simulink model "PA_PUC7_ThreeSystem"  (R2023b)
settings: Solver=ode23  StartTime=0.0  StopTime=7  MaxStep=1e-5  MinStep=1e-6  RelTol=1e-3
libraries: simulink x33, spsSeriesRLCBranchLib x30, spsIGBTDiodeLib x24, spsDiodeLib x21, dspstat3 x18, spsCurrentMeasurementLib x12, spsVoltageMeasurementLib x12, spsMosfetLib x9, spsVariableResistorLib x3, spsDCVoltageSourceLib x3, fuzblock x2, spspowerguiLib x1
settings Model: Creator=T5610  LastModifiedBy=afuaf
settings SolverCC: AlgebraicLoopSolver=TrustRegion
settings DataIOCC: ReturnWorkspaceOutputs=off
settings DebuggingCC: UnconnectedInputMsg=warning  UnconnectedOutputMsg=warning  UnconnectedLineMsg=warning
settings ModelReferenceCC: EnableRefExpFcnMdlSchedulingChecks=on

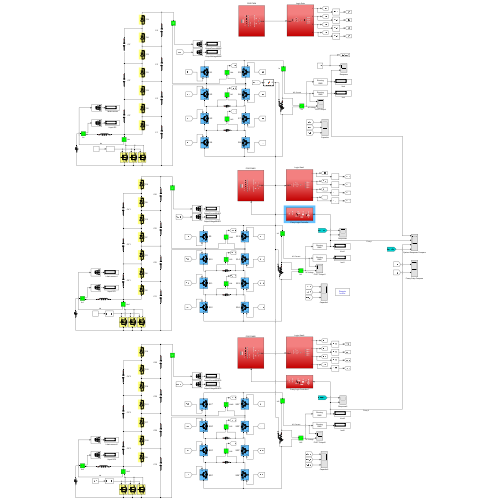
[thumbnail: Simulink's stored preview of the top-level diagram]
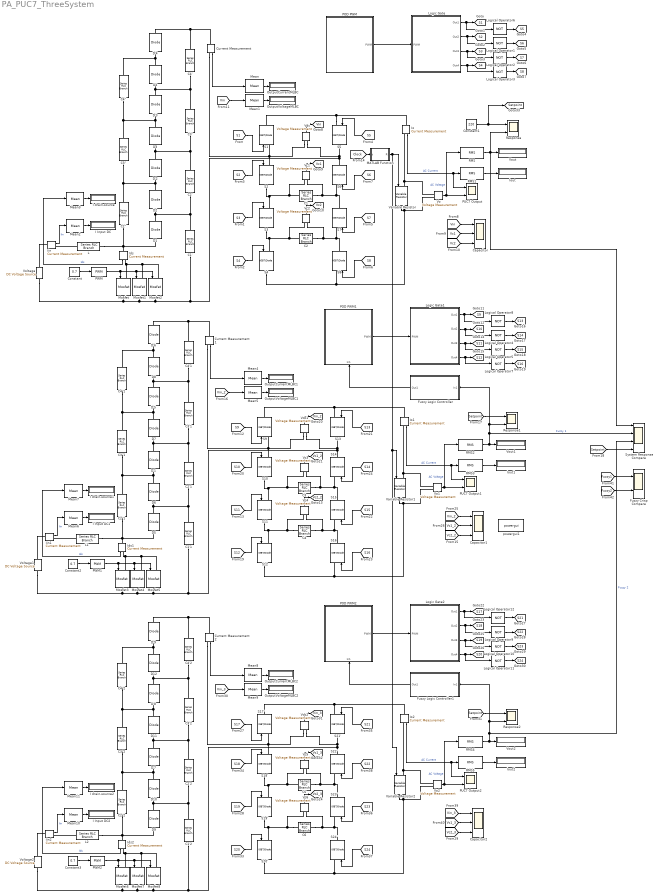
== system PA_PUC7_ThreeSystem ==
  C{1..6} (6 alike) : spsSeriesRLCBranchLib/Series RLC Branch  LConnTagsString=__new0  RConnTagsString=__new0  BranchType=C  Resistance=1  Inductance=100e-03  SetiL0=off  InitialCurrent=0  Capacitance=470e-6  Setx0=on  InitialVoltage=0  Measurements=None
  C1' : spsSeriesRLCBranchLib/Series RLC Branch  LConnTagsString=__new0  RConnTagsString=__new0  BranchType=C  Resistance=5e-3  Inductance=1e-3  SetiL0=off  InitialCurrent=0  Capacitance=3300e-6  Setx0=on  InitialVoltage=0  Measurements=None
  C1'1 : spsSeriesRLCBranchLib/Series RLC Branch  LConnTagsString=__new0  RConnTagsString=__new0  BranchType=C  Resistance=5e-3  Inductance=1e-3  SetiL0=off  InitialCurrent=0  Capacitance=3300e-6  Setx0=on  InitialVoltage=0  Measurements=None
  C1'2 : spsSeriesRLCBranchLib/Series RLC Branch  LConnTagsString=__new0  RConnTagsString=__new0  BranchType=C  Resistance=5e-3  Inductance=1e-3  SetiL0=off  InitialCurrent=0  Capacitance=3300e-6  Setx0=on  InitialVoltage=0  Measurements=None
  C2' : spsSeriesRLCBranchLib/Series RLC Branch  LConnTagsString=__new0  RConnTagsString=__new0  BranchType=C  Resistance=5e-3  Inductance=1e-3  SetiL0=off  InitialCurrent=0  Capacitance=3300e-6  Setx0=on  InitialVoltage=0  Measurements=None
  C2'' : spsSeriesRLCBranchLib/Series RLC Branch  LConnTagsString=__new0  RConnTagsString=__new0  BranchType=C  Resistance=5e-3  Inductance=1e-3  SetiL0=off  InitialCurrent=0  Capacitance=3300e-6  Setx0=on  InitialVoltage=0  Measurements=None
  C2''1 : spsSeriesRLCBranchLib/Series RLC Branch  LConnTagsString=__new0  RConnTagsString=__new0  BranchType=C  Resistance=5e-3  Inductance=1e-3  SetiL0=off  InitialCurrent=0  Capacitance=3300e-6  Setx0=on  InitialVoltage=0  Measurements=None
  C2''2 : spsSeriesRLCBranchLib/Series RLC Branch  LConnTagsString=__new0  RConnTagsString=__new0  BranchType=C  Resistance=5e-3  Inductance=1e-3  SetiL0=off  InitialCurrent=0  Capacitance=3300e-6  Setx0=on  InitialVoltage=0  Measurements=None
  C2'1 : spsSeriesRLCBranchLib/Series RLC Branch  LConnTagsString=__new0  RConnTagsString=__new0  BranchType=C  Resistance=5e-3  Inductance=1e-3  SetiL0=off  InitialCurrent=0  Capacitance=3300e-6  Setx0=on  InitialVoltage=0  Measurements=None
  C2'2 : spsSeriesRLCBranchLib/Series RLC Branch  LConnTagsString=__new0  RConnTagsString=__new0  BranchType=C  Resistance=5e-3  Inductance=1e-3  SetiL0=off  InitialCurrent=0  Capacitance=3300e-6  Setx0=on  InitialVoltage=0  Measurements=None
  C3' : spsSeriesRLCBranchLib/Series RLC Branch  LConnTagsString=__new0  RConnTagsString=__new0  BranchType=C  Resistance=5e-3  Inductance=1e-3  SetiL0=off  InitialCurrent=0  Capacitance=3300e-6  Setx0=on  InitialVoltage=0  Measurements=None
  C3'' : spsSeriesRLCBranchLib/Series RLC Branch  LConnTagsString=__new0  RConnTagsString=__new0  BranchType=C  Resistance=5e-3  Inductance=1e-3  SetiL0=off  InitialCurrent=0  Capacitance=3300e-6  Setx0=on  InitialVoltage=0  Measurements=None
  C3''1 : spsSeriesRLCBranchLib/Series RLC Branch  LConnTagsString=__new0  RConnTagsString=__new0  BranchType=C  Resistance=5e-3  Inductance=1e-3  SetiL0=off  InitialCurrent=0  Capacitance=3300e-6  Setx0=on  InitialVoltage=0  Measurements=None
  C3''2 : spsSeriesRLCBranchLib/Series RLC Branch  LConnTagsString=__new0  RConnTagsString=__new0  BranchType=C  Resistance=5e-3  Inductance=1e-3  SetiL0=off  InitialCurrent=0  Capacitance=3300e-6  Setx0=on  InitialVoltage=0  Measurements=None
  C3'1 : spsSeriesRLCBranchLib/Series RLC Branch  LConnTagsString=__new0  RConnTagsString=__new0  BranchType=C  Resistance=5e-3  Inductance=1e-3  SetiL0=off  InitialCurrent=0  Capacitance=3300e-6  Setx0=on  InitialVoltage=0  Measurements=None
  C3'2 : spsSeriesRLCBranchLib/Series RLC Branch  LConnTagsString=__new0  RConnTagsString=__new0  BranchType=C  Resistance=5e-3  Inductance=1e-3  SetiL0=off  InitialCurrent=0  Capacitance=3300e-6  Setx0=on  InitialVoltage=0  Measurements=None
  C4' : spsSeriesRLCBranchLib/Series RLC Branch  LConnTagsString=__new0  RConnTagsString=__new0  BranchType=C  Resistance=5e-3  Inductance=1e-3  SetiL0=off  InitialCurrent=0  Capacitance=3300e-6  Setx0=on  InitialVoltage=0  Measurements=None
  C4'' : spsSeriesRLCBranchLib/Series RLC Branch  LConnTagsString=__new0  RConnTagsString=__new0  BranchType=C  Resistance=5e-3  Inductance=1e-3  SetiL0=off  InitialCurrent=0  Capacitance=3300e-6  Setx0=on  InitialVoltage=0  Measurements=None
  C4''1 : spsSeriesRLCBranchLib/Series RLC Branch  LConnTagsString=__new0  RConnTagsString=__new0  BranchType=C  Resistance=5e-3  Inductance=1e-3  SetiL0=off  InitialCurrent=0  Capacitance=3300e-6  Setx0=on  InitialVoltage=0  Measurements=None
  C4''2 : spsSeriesRLCBranchLib/Series RLC Branch  LConnTagsString=__new0  RConnTagsString=__new0  BranchType=C  Resistance=5e-3  Inductance=1e-3  SetiL0=off  InitialCurrent=0  Capacitance=3300e-6  Setx0=on  InitialVoltage=0  Measurements=None
  C4'1 : spsSeriesRLCBranchLib/Series RLC Branch  LConnTagsString=__new0  RConnTagsString=__new0  BranchType=C  Resistance=5e-3  Inductance=1e-3  SetiL0=off  InitialCurrent=0  Capacitance=3300e-6  Setx0=on  InitialVoltage=0  Measurements=None
  C4'2 : spsSeriesRLCBranchLib/Series RLC Branch  LConnTagsString=__new0  RConnTagsString=__new0  BranchType=C  Resistance=5e-3  Inductance=1e-3  SetiL0=off  InitialCurrent=0  Capacitance=3300e-6  Setx0=on  InitialVoltage=0  Measurements=None
  Capacitor : Scope  NumInputPorts=3
  Capacitor1 : Scope  NumInputPorts=3
  Capacitor2 : Scope  NumInputPorts=3
  Constant : Constant  Value=0.7
  Constant1 : Constant  Value=220
  Constant2 : Constant  Value=0.7
  Constant3 : Constant  Value=0.7
  Current Measurement : spsCurrentMeasurementLib/Current Measurement  PhasorSimulation=off  OutputType=Complex  PSBequivalent=0
  Current Measurement1 : spsCurrentMeasurementLib/Current Measurement  PhasorSimulation=off  OutputType=Complex  PSBequivalent=0
  Current Measurement2 : spsCurrentMeasurementLib/Current Measurement  PhasorSimulation=off  OutputType=Complex  PSBequivalent=0
  D'{1..9} (9 alike) : spsDiodeLib/Diode  Ron=0.001  Lon=0  Vf=0.8  IC=0  UseSnubber=off  Rs=500  Cs=250e-9  Measurements=off
  D{1..12} (12 alike) : spsDiodeLib/Diode  Ron=0.001  Lon=0  Vf=0.8  IC=0  UseSnubber=off  Rs=500  Cs=250e-9  Measurements=off
  Fuzzy Crisp Compare : Scope  NumInputPorts=2
  Fuzzy Logic Controller : Subsystem
  Fuzzy Logic Controller1 : Subsystem
  I Input DC : Display
  I Input DC1 : Display
  I Input DC2 : Display
  I drain-source : Display
  I drain-source1 : Display
  I drain-source2 : Display
  Ids : spsCurrentMeasurementLib/Current Measurement  Tag=PoWeRsYsTeMmEaSuReMeNt  PhasorSimulation=off  OutputType=Magnitude  PSBequivalent=0
      settings: AttributesFormatString=\n
  Ids1 : spsCurrentMeasurementLib/Current Measurement  Tag=PoWeRsYsTeMmEaSuReMeNt  PhasorSimulation=off  OutputType=Magnitude  PSBequivalent=0
      settings: AttributesFormatString=\n
  Ids2 : spsCurrentMeasurementLib/Current Measurement  Tag=PoWeRsYsTeMmEaSuReMeNt  PhasorSimulation=off  OutputType=Magnitude  PSBequivalent=0
      settings: AttributesFormatString=\n
  Iin : spsCurrentMeasurementLib/Current Measurement  Tag=PoWeRsYsTeMmEaSuReMeNt  PhasorSimulation=off  OutputType=Magnitude  PSBequivalent=0
      settings: AttributesFormatString=\n
  Iin1 : spsCurrentMeasurementLib/Current Measurement  Tag=PoWeRsYsTeMmEaSuReMeNt  PhasorSimulation=off  OutputType=Magnitude  PSBequivalent=0
      settings: AttributesFormatString=\n
  Iin2 : spsCurrentMeasurementLib/Current Measurement  Tag=PoWeRsYsTeMmEaSuReMeNt  PhasorSimulation=off  OutputType=Magnitude  PSBequivalent=0
      settings: AttributesFormatString=\n
  Io : spsCurrentMeasurementLib/Current Measurement  Tag=PoWeRsYsTeMmEaSuReMeNt  PhasorSimulation=off  OutputType=Magnitude  PSBequivalent=0
      settings: AttributesFormatString=\n
  Io1 : spsCurrentMeasurementLib/Current Measurement  Tag=PoWeRsYsTeMmEaSuReMeNt  PhasorSimulation=off  OutputType=Magnitude  PSBequivalent=0
      settings: AttributesFormatString=\n
  Io2 : spsCurrentMeasurementLib/Current Measurement  Tag=PoWeRsYsTeMmEaSuReMeNt  PhasorSimulation=off  OutputType=Magnitude  PSBequivalent=0
      settings: AttributesFormatString=\n
  Iout : Display
  Iout1 : Display
  Iout2 : Display
  L : spsSeriesRLCBranchLib/Series RLC Branch  LConnTagsString=__new0  RConnTagsString=__new0  BranchType=L  Resistance=0.5  Inductance=76.289e-6  SetiL0=on  InitialCurrent=0  Capacitance=1e-6  Setx0=off  InitialVoltage=0  Measurements=None
  L1 : spsSeriesRLCBranchLib/Series RLC Branch  LConnTagsString=__new0  RConnTagsString=__new0  BranchType=L  Resistance=0.5  Inductance=76.289e-6  SetiL0=on  InitialCurrent=0  Capacitance=1e-6  Setx0=off  InitialVoltage=0  Measurements=None
  L2 : spsSeriesRLCBranchLib/Series RLC Branch  LConnTagsString=__new0  RConnTagsString=__new0  BranchType=L  Resistance=0.5  Inductance=76.289e-6  SetiL0=on  InitialCurrent=0  Capacitance=1e-6  Setx0=off  InitialVoltage=0  Measurements=None
  Logic Gate : Subsystem
  Logic Gate1 : Subsystem
  Logic Gate2 : Subsystem
  Logical Operator{1..12} (12 alike) : Logic  Operator=NOT  Inputs=3  AllPortsSameDT=off  OutDataTypeStr=boolean
  MATLAB Function : MATLAB Function  TreatAsAtomicUnit=on
  Mean{,1..11} (12 alike) : dspstat3/Mean  run=on  InputProcessing=Columns as channels (frame based)  reset_popup=None  directionMode=Each column  dimension=1  roiEnable=off  roiType=Rectangles  roiPortion=Entire ROI  roiOutput=Individual statistics for each ROI  roiFlag=off  roundingMode=Floor  overflowMode=off  outputDataTypeStr=Inherit: Same as accumulator  outputMin=[]  outputMax=[]  outputLastDataTypeStr=Inherit: Same as accumulator
  Mosfet{,1..8} (9 alike) : spsMosfetLib/Mosfet  Ron=0.1  Lon=0  Rd=0.01  Vfd=0  IC=0  Rs=4700  Cs=1.8e-9  Measurements=off
  OutputCurrentMLBC : Display
  OutputCurrentMLBC1 : Display
  OutputCurrentMLBC2 : Display
  OutputVoltageMLBC : Display
  OutputVoltageMLBC1 : Display
  OutputVoltageMLBC2 : Display
  POD PWM : Subsystem
  POD PWM1 : Subsystem
      settings: PortSchema="{\"entries\":[{\"content\":{\"sides\":[{\"content\":{},\"type\":\"ConnectorPlacement.EquallySpacedRectSide\",\"uuid\":\"fc441c86-3ac2-46d8-9061-132decdd35e5\"},{\"content\":{\"connectorIds\":[\"Out1\"],\"side\":\"RIGHT\"},\"type\":\"ConnectorPlacement.EquallySpacedRectSide\",\"uuid\":\"7d69d47a-a4f5-4f75-a9c0-214fc8de94d4\"},{\"content\":{\"side\":\"TOP\"},\"type\":\"ConnectorPlacement.EquallySpacedRectSide\",\"uuid\":\"70f1275d-73bb-4298-b141-4f36cf048c09\"},{\"content\":{\"connectorIds\":[\"In1\"],\"side\":\"BOTTOM\"},\"type\":\"ConnectorPlacement.EquallySpacedRectSide\",\"uuid\":\"f86154e3-f7e3-4243-8b55-8a0e53d9a2a3\"}]},\"type\":\"ConnectorPlacement.EquallySpacedConnector\",\"uuid\":\"5fb14212-564c-4c50-825a-0041235b0c9e\"}],\"packageUris\":[\"http://schema.mathworks.com/mf0/Connector/R2020b\"],\"version\":\"1.0\"}"
  POD PWM2 : Subsystem
      settings: PortSchema="{\"entries\":[{\"content\":{\"sides\":[{\"content\":{},\"type\":\"ConnectorPlacement.EquallySpacedRectSide\",\"uuid\":\"fc441c86-3ac2-46d8-9061-132decdd35e5\"},{\"content\":{\"connectorIds\":[\"Out1\"],\"side\":\"RIGHT\"},\"type\":\"ConnectorPlacement.EquallySpacedRectSide\",\"uuid\":\"7d69d47a-a4f5-4f75-a9c0-214fc8de94d4\"},{\"content\":{\"side\":\"TOP\"},\"type\":\"ConnectorPlacement.EquallySpacedRectSide\",\"uuid\":\"70f1275d-73bb-4298-b141-4f36cf048c09\"},{\"content\":{\"connectorIds\":[\"In1\"],\"side\":\"BOTTOM\"},\"type\":\"ConnectorPlacement.EquallySpacedRectSide\",\"uuid\":\"f86154e3-f7e3-4243-8b55-8a0e53d9a2a3\"}]},\"type\":\"ConnectorPlacement.EquallySpacedConnector\",\"uuid\":\"5fb14212-564c-4c50-825a-0041235b0c9e\"}],\"packageUris\":[\"http://schema.mathworks.com/mf0/Connector/R2020b\"],\"version\":\"1.0\"}"
  PUC7 Output : Scope  NumInputPorts=2
  PUC7 Output1 : Scope  NumInputPorts=2
  PUC7 Output2 : Scope  NumInputPorts=2
  PWM : simulink/Discontinuities/PWM  DisableCoverage=on  Period=1/40000  InitialDelay=0  DisallowZeroDutyCycle=off  RunAtFixedTimeIntervals=off  SampleTime=0.1
  PWM1 : simulink/Discontinuities/PWM  DisableCoverage=on  Period=1/40000  InitialDelay=0  DisallowZeroDutyCycle=off  RunAtFixedTimeIntervals=off  SampleTime=0.1
  PWM2 : simulink/Discontinuities/PWM  DisableCoverage=on  Period=1/40000  InitialDelay=0  DisallowZeroDutyCycle=off  RunAtFixedTimeIntervals=off  SampleTime=0.1
  RMS{,1..5} (6 alike) : dspstat3/RMS  run=on  directionMode=Each column  dimension=1  InputProcessing=Columns as channels (frame based)  reset_popup=None
  Response : Scope  NumInputPorts=2
  Response1 : Scope  NumInputPorts=2
  Response2 : Scope  NumInputPorts=2
  S{1..16} (16 alike) : spsIGBTDiodeLib/IGBT//Diode  Ron=1e-3  Rs=1e5  Cs=inf  Measurements=off
  S17' : spsIGBTDiodeLib/IGBT//Diode  Ron=1e-3  Rs=1e5  Cs=inf  Measurements=off
  S18' : spsIGBTDiodeLib/IGBT//Diode  Ron=1e-3  Rs=1e5  Cs=inf  Measurements=off
  S19' : spsIGBTDiodeLib/IGBT//Diode  Ron=1e-3  Rs=1e5  Cs=inf  Measurements=off
  S20' : spsIGBTDiodeLib/IGBT//Diode  Ron=1e-3  Rs=1e5  Cs=inf  Measurements=off
  S21' : spsIGBTDiodeLib/IGBT//Diode  Ron=1e-3  Rs=1e5  Cs=inf  Measurements=off
  S22' : spsIGBTDiodeLib/IGBT//Diode  Ron=1e-3  Rs=1e5  Cs=inf  Measurements=off
  S23' : spsIGBTDiodeLib/IGBT//Diode  Ron=1e-3  Rs=1e5  Cs=inf  Measurements=off
  S24' : spsIGBTDiodeLib/IGBT//Diode  Ron=1e-3  Rs=1e5  Cs=inf  Measurements=off
  System Response Compare : Scope  NumInputPorts=4
  Variable Resistor : spsVariableResistorLib/Variable Resistor  Rabsmin=1e-3
      settings: LibrarySourceBlock=sps_lib/Passives/Variable Resistor
  Variable Resistor1 : spsVariableResistorLib/Variable Resistor  Rabsmin=1e-3
      settings: LibrarySourceBlock=sps_lib/Passives/Variable Resistor
  Variable Resistor2 : spsVariableResistorLib/Variable Resistor  Rabsmin=1e-3
      settings: LibrarySourceBlock=sps_lib/Passives/Variable Resistor
  Vc{1..6} (6 alike) : spsVoltageMeasurementLib/Voltage Measurement  Tag=PoWeRsYsTeMmEaSuReMeNt  PhasorSimulation=off  OutputType=Magnitude  PSBequivalent=0
  Vdc : spsVoltageMeasurementLib/Voltage Measurement  Tag=PoWeRsYsTeMmEaSuReMeNt  PhasorSimulation=off  OutputType=Magnitude  PSBequivalent=0
  Vdc1 : spsVoltageMeasurementLib/Voltage Measurement  Tag=PoWeRsYsTeMmEaSuReMeNt  PhasorSimulation=off  OutputType=Magnitude  PSBequivalent=0
  Vdc2 : spsVoltageMeasurementLib/Voltage Measurement  Tag=PoWeRsYsTeMmEaSuReMeNt  PhasorSimulation=off  OutputType=Magnitude  PSBequivalent=0
  Vo : spsVoltageMeasurementLib/Voltage Measurement  Tag=PoWeRsYsTeMmEaSuReMeNt  PhasorSimulation=off  OutputType=Magnitude  PSBequivalent=0
  Vo1 : spsVoltageMeasurementLib/Voltage Measurement  Tag=PoWeRsYsTeMmEaSuReMeNt  PhasorSimulation=off  OutputType=Magnitude  PSBequivalent=0
  Vo2 : spsVoltageMeasurementLib/Voltage Measurement  Tag=PoWeRsYsTeMmEaSuReMeNt  PhasorSimulation=off  OutputType=Magnitude  PSBequivalent=0
  Voltage : spsDCVoltageSourceLib/DC Voltage Source  Amplitude=24  Measurements=None
  Voltage1 : spsDCVoltageSourceLib/DC Voltage Source  Amplitude=24  Measurements=None
  Voltage2 : spsDCVoltageSourceLib/DC Voltage Source  Amplitude=24  Measurements=None
  Vout : Display
  Vout1 : Display
  Vout2 : Display
  powergui1 : spspowerguiLib/powergui  Priority=1  SimulationMode=Discrete  SampleTime=1e-6  frequency=50  Iterations=50  frequencyindice=0  Pbase=100e6  ErrMax=1e-4  UnitsV=kV  UnitsW=MW  buscounter=0  FunctionMessages=off  echomessages=off  EnableUseOfTLC=off  CurrentSourceSwitches=off  DisableSnubberDevices=off  DisableRonSwitches=off  DisableVfSwitches=off  DisplayEquations=off  AutomaticDiscreteSolvers=off  SolverType=Tustin/Backward Euler (TBE)  Interpol=off  ExternalGateDelay=off  methode=off  Ts=100  x0status=blocks  SPID=on  SwTol=0  HookPort=off  NonlinearTolerance=1e-4  nMaxIteration=100  ContinueOnMaxIteration=off  RestoreLinks=warning  ResistiveCurrentMeasurement=off  Frange=[0:2:500]  Ylog=off  Xlog=on  ShowGrid=off  save=off  variable=ZData  structure=PUC_Output  ZoomFFT=off  StartTime=3  cycles=1  DisplayStyle=1  fundamental=50  FreqAxis=on  MaxFrequency=1000  frequencyindicesteady=1  RmsSteady=1  display=off
  tag scope: S10=global, S11=global, S12=global, S13=global, S14=global, S15=global, S16=global, S17=global, S18=global, S19=global, S1=global, S20=global, S21=global, S22=global, S23=global, S24=global, S2=global, S3=global, S4=global, S5=global, S6=global, S7=global, S8=global, S9=global, Setpoint=global, Vc1=global, Vc1_2=global, Vc1_3=global, Vc2=global, Vc2_2=global, Vc2_3=global, Vin=global, Vin_2=global, Vin_3=global
  wires:
  POD PWM/1(PWM) -> Logic Gate/1(PWM)
  [S5] -> S5/1
  Vo/1 -> RMS/1, PUC7 Output/2  "AC Voltage"
  [S1] -> S1/1
  [S2] -> S2/1
  [S6] -> S6/1
  [S3] -> S3/1
  [S7] -> S7/1
  [S8] -> S8/1
  [S4] -> S4/1
  Logical Operator6/1 -> [S5]
  Logic Gate/1(Out1) -> [S1], Logical Operator6/1
  Logic Gate/2(Out2) -> [S2], Logical Operator1/1
  Logical Operator1/1 -> [S6]
  Logic Gate/3(Out3) -> [S3], Logical Operator2/1
  Logical Operator2/1 -> [S7]
  Logic Gate/4(Out4) -> [S4], Logical Operator3/1
  Logical Operator3/1 -> [S8]
  RMS/1 -> System Response Compare/1, Vout/1, Response/2
  RMS1/1 -> Iout/1
  Constant/1 -> PWM/1
  Current Measurement/1 -> Mean/1
  Vdc/1 -> [Vin]
  Vc1/1 -> [Vc1]
  Vc2/1 -> [Vc2]
  [Vin] -> Capacitor/1
  [Vc1] -> Capacitor/2
  [Vc2] -> Capacitor/3
  Mean/1 -> OutputCurrentMLBC/1
  Mean1/1 -> OutputVoltageMLBC/1
  [Vin] -> Mean1/1
  Mean2/1 -> I Input DC/1
  Iin/1 -> Mean2/1  "Iin"
  Mean3/1 -> I drain-source/1
  Ids/1 -> Mean3/1  "Ids"
  PWM/1 -> Mosfet/1, Mosfet1/1, Mosfet2/1
  Io/1 -> PUC7 Output/1, RMS1/1  "AC Current"
  MATLAB Function/1(R) -> Variable Resistor2/1, Variable Resistor1/1, Variable Resistor/1
  [Clock] -> MATLAB Function/1(t)
  Constant1/1 -> [Setpoint], Response/1
  Fuzzy Logic Controller/1(Out1) -> POD PWM1/1(In1)
  [Setpoint] -> Response1/1
  RMS3/1 -> Iout1/1
  [S16] -> S16/1
  Logical Operator4/1 -> [S14]
  RMS2/1 -> Response1/2, Fuzzy Logic Controller/1(In1), System Response Compare/2, Vout1/1  "Fuzzy 1"
  Logical Operator7/1 -> [S16]
  Logical Operator5/1 -> [S15]
  [S14] -> S14/1
  Logic Gate1/1(Out1) -> [S9], Logical Operator8/1
  [S15] -> S15/1
  Logical Operator8/1 -> [S13]
  POD PWM1/1(PWM) -> Logic Gate1/1(PWM)
  [S13] -> S13/1
  Vo1/1 -> RMS2/1, PUC7 Output1/2  "AC Voltage"
  Vc4/1 -> [Vc2_2]
  [Vin_2] -> Capacitor1/1
  [S10] -> S10/1
  [Vc2_2] -> Capacitor1/3
  Vdc1/1 -> [Vin_2]
  Mean4/1 -> OutputCurrentMLBC1/1
  [Vin_2] -> Mean5/1
  [S12] -> S12/1
  Constant2/1 -> PWM1/1
  Current Measurement1/1 -> Mean4/1
  Logic Gate1/4(Out4) -> [S12], Logical Operator7/1
  PWM1/1 -> Mosfet3/1, Mosfet4/1, Mosfet5/1
  Mean5/1 -> OutputVoltageMLBC1/1
  Iin1/1 -> Mean6/1  "Iin"
  [S9] -> S9/1
  Logic Gate1/2(Out2) -> [S10], Logical Operator4/1
  Mean7/1 -> I drain-source1/1
  [S11] -> S11/1
  Io1/1 -> PUC7 Output1/1, RMS3/1  "AC Current"
  [Vc1_2] -> Capacitor1/2
  Ids1/1 -> Mean7/1  "Ids"
  Vc3/1 -> [Vc1_2]
  Mean6/1 -> I Input DC1/1
  Logic Gate1/3(Out3) -> [S11], Logical Operator5/1
  Mean10/1 -> I Input DC2/1
  Vc5/1 -> [Vc1_3]
  Logic Gate2/3(Out3) -> [S19], Logical Operator10/1
  Ids2/1 -> Mean11/1  "Ids"
  Vc6/1 -> [Vc2_3]
  Vdc2/1 -> [Vin_3]
  [Vc2_3] -> Capacitor2/3
  Mean8/1 -> OutputCurrentMLBC2/1
  Logical Operator10/1 -> [S23]
  [S22] -> S22'/1
  [S21] -> S21'/1
  RMS4/1 -> System Response Compare/3, Response2/2, Fuzzy Logic Controller1/1(In1), Vout2/1  "Fuzzy 2"
  Vo2/1 -> RMS4/1, PUC7 Output2/2  "AC Voltage"
  POD PWM2/1(PWM) -> Logic Gate2/1(PWM)
  Logical Operator11/1 -> [S24]
  Logic Gate2/1(Out1) -> [S17], Logical Operator12/1
  Logical Operator12/1 -> [S21]
  RMS5/1 -> Iout2/1
  [S18] -> S18'/1
  Logical Operator9/1 -> [S22]
  [S24] -> S24'/1
  [Setpoint] -> Response2/1
  Fuzzy Logic Controller1/1(Out1) -> POD PWM2/1(In1)
  [Vc1_3] -> Capacitor2/2
  Mean11/1 -> I drain-source2/1
  Iin2/1 -> Mean10/1  "Iin"
  Logic Gate2/2(Out2) -> [S18], Logical Operator9/1
  [S19] -> S19'/1
  [S17] -> S17'/1
  [S20] -> S20'/1
  [Vin_3] -> Mean9/1
  Mean9/1 -> OutputVoltageMLBC2/1
  Current Measurement2/1 -> Mean8/1
  Constant3/1 -> PWM2/1
  [Vin_3] -> Capacitor2/1
  PWM2/1 -> Mosfet6/1, Mosfet7/1, Mosfet8/1
  [S23] -> S23'/1
  Io2/1 -> PUC7 Output2/1, RMS5/1  "AC Current"
  Logic Gate2/4(Out4) -> [S20], Logical Operator11/1
  [Fuzzy1] -> Fuzzy Crisp Compare/1
  [Fuzzy2] -> Fuzzy Crisp Compare/2
  [Setpoint] -> System Response Compare/4
  connections:
  S5/LConn1 -- Io/LConn1 -- S1/RConn1
  Vo/LConn1 -- Variable Resistor/LConn1 -- Io/RConn1
  Vdc/LConn1 -- Current Measurement/RConn1 -- S2/LConn1 -- S1/LConn1
  S2/RConn1 -- C1/LConn1 -- Vc1/LConn1 -- S3/LConn1
  C1/RConn1 -- Vc1/LConn2 -- S7/RConn1 -- S6/LConn1
  S3/RConn1 -- S4/LConn1 -- Vc2/LConn1 -- C2/LConn1
  C2/RConn1 -- Vc2/LConn2 -- S8/RConn1 -- S7/LConn1
  S4/RConn1 -- Variable Resistor/RConn1 -- Vo/LConn2 -- S8/LConn1
  D4/LConn1 -- D'3/RConn1 -- C4'/RConn1 -- C3'/LConn1
  D'2/LConn1 -- D2/RConn1 -- C2''/LConn1 -- C3''/RConn1
  D2/LConn1 -- D1/RConn1 -- C1'/LConn1 -- C2'/RConn1
  C4''/RConn1 -- D3/RConn1 -- D'3/LConn1 -- C3''/LConn1
  C2''/RConn1 -- Ids/LConn1 -- L/RConn1 -- D1/LConn1
  Vdc/LConn2 -- S6/RConn1 -- C1'/RConn1 -- Voltage/LConn1 -- Mosfet/RConn1 -- Mosfet1/RConn1 -- Mosfet2/RConn1 -- S5/RConn1
  D'4/RConn1 -- C4'/LConn1 -- Current Measurement/LConn1
  C2'/LConn1 -- D'2/RConn1 -- D3/LConn1 -- C3'/RConn1
  D'4/LConn1 -- D4/RConn1 -- C4''/LConn1
  L/LConn1 -- Iin/RConn1
  Voltage/RConn1 -- Iin/LConn1
  Ids/RConn1 -- Mosfet2/LConn1 -- Mosfet1/LConn1 -- Mosfet/LConn1
  C3''1/RConn1 -- D'1/LConn1 -- D6/RConn1 -- C2''1/LConn1
  C3'1/LConn1 -- C4'1/RConn1 -- D8/LConn1 -- D'5/RConn1
  S9/LConn1 -- Vdc1/LConn1 -- Current Measurement1/RConn1 -- S10/LConn1
  Io1/RConn1 -- Vo1/LConn1 -- Variable Resistor1/LConn1
  S14/LConn1 -- C3/RConn1 -- Vc3/LConn2 -- S15/RConn1
  C3''1/LConn1 -- C4''1/RConn1 -- D7/RConn1 -- D'5/LConn1
  C4/LConn1 -- Vc4/LConn1 -- S11/RConn1 -- S12/LConn1
  S16/LConn1 -- S12/RConn1 -- Variable Resistor1/RConn1 -- Vo1/LConn2
  S13/RConn1 -- Vdc1/LConn2 -- S14/RConn1 -- C1'1/RConn1 -- Voltage1/LConn1 -- Mosfet3/RConn1 -- Mosfet4/RConn1 -- Mosfet5/RConn1
  S9/RConn1 -- S13/LConn1 -- Io1/LConn1
  Vc3/LConn1 -- S10/RConn1 -- S11/LConn1 -- C3/LConn1
  Mosfet4/LConn1 -- Ids1/RConn1 -- Mosfet3/LConn1 -- Mosfet5/LConn1
  D7/LConn1 -- C2'1/LConn1 -- C3'1/RConn1 -- D'1/RConn1
  D5/LConn1 -- C2''1/RConn1 -- Ids1/LConn1 -- L1/RConn1
  S15/LConn1 -- S16/RConn1 -- C4/RConn1 -- Vc4/LConn2
  Current Measurement1/LConn1 -- D'6/RConn1 -- C4'1/LConn1
  C2'1/RConn1 -- D6/LConn1 -- D5/RConn1 -- C1'1/LConn1
  C4''1/LConn1 -- D'6/LConn1 -- D8/RConn1
  L1/LConn1 -- Iin1/RConn1
  Voltage1/RConn1 -- Iin1/LConn1
  Current Measurement2/LConn1 -- D'9/RConn1 -- C4'2/LConn1
  D11/LConn1 -- C2'2/LConn1 -- C3'2/RConn1 -- D'7/RConn1
  Mosfet7/LConn1 -- Ids2/RConn1 -- Mosfet6/LConn1 -- Mosfet8/LConn1
  S21'/RConn1 -- Vdc2/LConn2 -- S22'/RConn1 -- C1'2/RConn1 -- Voltage2/LConn1 -- Mosfet6/RConn1 -- Mosfet7/RConn1 -- Mosfet8/RConn1
  C6/LConn1 -- Vc6/LConn1 -- S19'/RConn1 -- S20'/LConn1
  C3''2/RConn1 -- D'7/LConn1 -- D10/RConn1 -- C2''2/LConn1
  S24'/LConn1 -- S20'/RConn1 -- Variable Resistor2/RConn1 -- Vo2/LConn2
  S17'/RConn1 -- S21'/LConn1 -- Io2/LConn1
  C3''2/LConn1 -- C4''2/RConn1 -- D11/RConn1 -- D'8/LConn1
  S22'/LConn1 -- S23'/RConn1 -- C5/RConn1 -- Vc5/LConn2
  C2'2/RConn1 -- C1'2/LConn1 -- D10/LConn1 -- D9/RConn1
  C4''2/LConn1 -- D'9/LConn1 -- D12/RConn1
  Io2/RConn1 -- Vo2/LConn1 -- Variable Resistor2/LConn1
  S17'/LConn1 -- Vdc2/LConn1 -- Current Measurement2/RConn1 -- S18'/LConn1
  Vc5/LConn1 -- S18'/RConn1 -- S19'/LConn1 -- C5/LConn1
  C3'2/LConn1 -- C4'2/RConn1 -- D12/LConn1 -- D'8/RConn1
  S23'/LConn1 -- S24'/RConn1 -- C6/RConn1 -- Vc6/LConn2
  D9/LConn1 -- C2''2/RConn1 -- Ids2/LConn1 -- L2/RConn1
  Voltage2/RConn1 -- Iin2/LConn1
  L2/LConn1 -- Iin2/RConn1

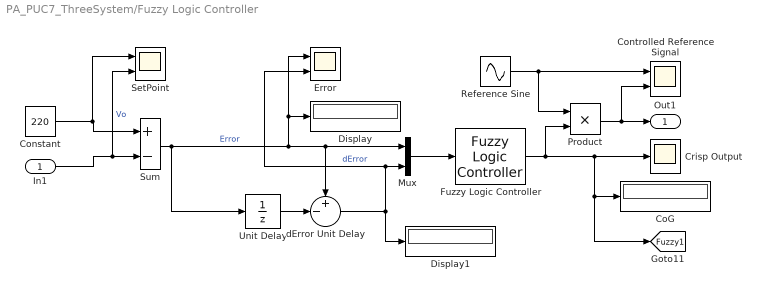
== system PA_PUC7_ThreeSystem/Fuzzy Logic Controller ==
  In1 : Inport
  CoG : Display
  Constant : Constant  Value=220
  Controlled Reference Signal : Scope  NumInputPorts=2
  Crisp Output : Scope
  Display : Display
  Display1 : Display
  Error : Scope  NumInputPorts=2
  Fuzzy Logic Controller : fuzblock/Fuzzy Logic  Controller  FIS=FuzzyType1_PA1_FIX  OutputSampleNumber=101  DataType=double  FuzzifiedInputs=off  RuleFiringStrengths=off  RuleOutputs=off  AggregatedOutputs=off  SimulateUsing=Interpreted execution  OutOfRangeInputValueMessage=none  NoRuleFiredMessage=none  EmptyOutputFuzzySetMessage=none
  Mux : Mux  Inputs=2
  Product : Product
  Reference Sine : Sin  Amplitude=3  Frequency=2*pi*50  Phase=2*pi*(3/4)  SampleTime=0
  SetPoint : Scope  NumInputPorts=2
  Sum : Sum  Inputs=+-
  Unit Delay : UnitDelay  SampleTime=-1  HasFrameUpgradeWarning=on
  dError Unit Delay : Sum  Inputs=+-|
  Out1 : Outport
  tag scope: Fuzzy1=global
  wires:
  In1/1 -> SetPoint/2, Sum/2  "Vo"
  Constant/1 -> SetPoint/1, Sum/1
  Sum/1 -> Unit Delay/1, Error/1, Display/1, Mux/1, dError Unit Delay/1  "Error"
  Mux/1 -> Fuzzy Logic Controller/1
  Reference Sine/1 -> Product/1, Controlled Reference Signal/1
  Fuzzy Logic Controller/1 -> [Fuzzy1], CoG/1, Crisp Output/1, Product/2
  Unit Delay/1 -> dError Unit Delay/2
  dError Unit Delay/1 -> Display1/1, Mux/2, Error/2  "dError"
  Product/1 -> Controlled Reference Signal/2, Out1/1

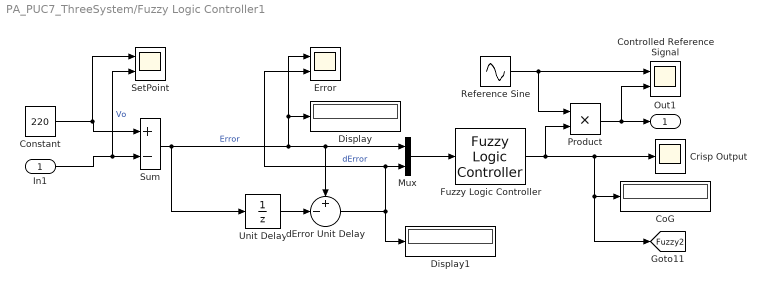
== system PA_PUC7_ThreeSystem/Fuzzy Logic Controller1 ==
  In1 : Inport
  CoG : Display
  Constant : Constant  Value=220
  Controlled Reference Signal : Scope  NumInputPorts=2
  Crisp Output : Scope
  Display : Display
  Display1 : Display
  Error : Scope  NumInputPorts=2
  Fuzzy Logic Controller : fuzblock/Fuzzy Logic  Controller  FIS=FuzzyType2_PA1_FIX  OutputSampleNumber=101  DataType=double  FuzzifiedInputs=off  RuleFiringStrengths=off  RuleOutputs=off  AggregatedOutputs=off  SimulateUsing=Interpreted execution  OutOfRangeInputValueMessage=none  NoRuleFiredMessage=none  EmptyOutputFuzzySetMessage=none
  Mux : Mux  Inputs=2
  Product : Product
  Reference Sine : Sin  Amplitude=3  Frequency=2*pi*50  Phase=2*pi*(3/4)  SampleTime=0
  SetPoint : Scope  NumInputPorts=2
  Sum : Sum  Inputs=+-
  Unit Delay : UnitDelay  SampleTime=-1  HasFrameUpgradeWarning=on
  dError Unit Delay : Sum  Inputs=+-|
  Out1 : Outport
  tag scope: Fuzzy2=global
  wires:
  In1/1 -> SetPoint/2, Sum/2  "Vo"
  Constant/1 -> SetPoint/1, Sum/1
  Sum/1 -> Unit Delay/1, Error/1, Display/1, Mux/1, dError Unit Delay/1  "Error"
  Mux/1 -> Fuzzy Logic Controller/1
  Reference Sine/1 -> Product/1, Controlled Reference Signal/1
  Fuzzy Logic Controller/1 -> CoG/1, [Fuzzy2], Crisp Output/1, Product/2
  Unit Delay/1 -> dError Unit Delay/2
  dError Unit Delay/1 -> Display1/1, Mux/2, Error/2  "dError"
  Product/1 -> Controlled Reference Signal/2, Out1/1

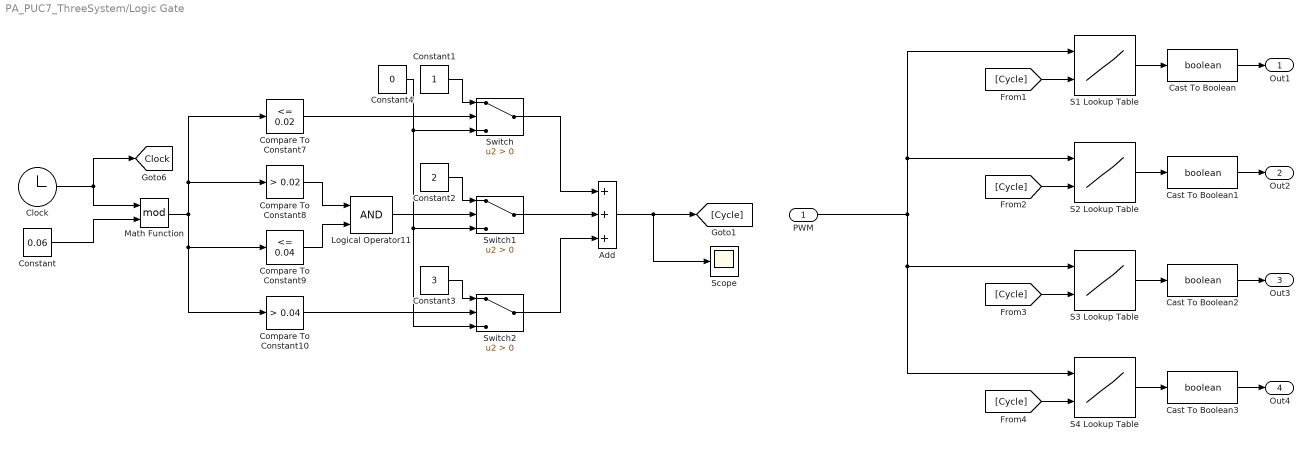
== system PA_PUC7_ThreeSystem/Logic Gate ==
  PWM : Inport
  Add : Sum  Inputs=+++
  Cast To Boolean{,1..3} (4 alike) : DataTypeConversion  OutDataTypeStr=boolean  SaturateOnIntegerOverflow=off  RndMeth=Floor
  Clock : Clock
  Compare To Constant10 : simulink/Logic and Bit Operations/Compare To Constant  relop=>  const=0.04  OutDataTypeStr=boolean
  Compare To Constant7 : simulink/Logic and Bit Operations/Compare To Constant  relop=<=  const=0.02  OutDataTypeStr=boolean
  Compare To Constant8 : simulink/Logic and Bit Operations/Compare To Constant  relop=>  const=0.02  OutDataTypeStr=boolean
  Compare To Constant9 : simulink/Logic and Bit Operations/Compare To Constant  relop=<=  const=0.04  OutDataTypeStr=boolean
  Constant : Constant  Value=0.06
  Constant1 : Constant
  Constant2 : Constant  Value=2
  Constant3 : Constant  Value=3
  Constant4 : Constant  Value=0
  Logical Operator11 : Logic  AllPortsSameDT=off  OutDataTypeStr=boolean
  Math Function : Math  Operator=mod
  S1 Lookup Table : Lookup_n-D  BreakpointsForDimension1=[-3:3]  BreakpointsForDimension2=[1:3]  Table=[0 0 0;0 0 0;0 0 0;1 0 1;1 1 1;1 1 1;1 1 1]  InternalRulePriority=Speed  RndMeth=Simplest
      settings: InputPortMap=u0,u1
  S2 Lookup Table : Lookup_n-D  BreakpointsForDimension1=[-3:3]  BreakpointsForDimension2=[1:3]  Table=[1 1 1;1 0 1;1 0 0;1 0 1;0 1 1;0 1 0;0 0 0]  InternalRulePriority=Speed  RndMeth=Simplest
      settings: InputPortMap=u0,u1
  S3 Lookup Table : Lookup_n-D  BreakpointsForDimension1=[-3:3]  BreakpointsForDimension2=[1:3]  Table=[1 1 1;0 1 1;0 1 0;1 0 1;1 0 1;1 0 0;0 0 0]  InternalRulePriority=Speed  RndMeth=Simplest
      settings: InputPortMap=u0,u1
  S4 Lookup Table : Lookup_n-D  BreakpointsForDimension1=[-3:3]  BreakpointsForDimension2=[1:3]  Table=[1 1 1;1 1 0;0 0 1;1 0 1;1 1 0;0 0 1;0 0 0]  InternalRulePriority=Speed  RndMeth=Simplest
      settings: InputPortMap=u0,u1
  Scope : Scope
  Switch : Switch  Criteria=u2 > Threshold  SaturateOnIntegerOverflow=off  InputSameDT=off
  Switch1 : Switch  Criteria=u2 > Threshold  SaturateOnIntegerOverflow=off  InputSameDT=off
  Switch2 : Switch  Criteria=u2 > Threshold  SaturateOnIntegerOverflow=off  InputSameDT=off
  Out1 : Outport
  Out2 : Outport  Port=2
  Out3 : Outport  Port=3
  Out4 : Outport  Port=4
  tag scope: Clock=global
  wires:
  Clock/1 -> Math Function/1, [Clock]
  Constant/1 -> Math Function/2
  Math Function/1 -> Compare To Constant7/1, Compare To Constant8/1, Compare To Constant9/1, Compare To Constant10/1
  Compare To Constant8/1 -> Logical Operator11/1
  Compare To Constant9/1 -> Logical Operator11/2
  S1 Lookup Table/1 -> Cast To Boolean/1
  S2 Lookup Table/1 -> Cast To Boolean1/1
  S3 Lookup Table/1 -> Cast To Boolean2/1
  S4 Lookup Table/1 -> Cast To Boolean3/1
  Compare To Constant7/1 -> Switch/2
  Logical Operator11/1 -> Switch1/2
  Constant1/1 -> Switch/1
  Constant2/1 -> Switch1/1
  Constant3/1 -> Switch2/1
  Compare To Constant10/1 -> Switch2/2
  [Cycle] -> S1 Lookup Table/2
  [Cycle] -> S2 Lookup Table/2
  [Cycle] -> S3 Lookup Table/2
  [Cycle] -> S4 Lookup Table/2
  PWM/1 -> S4 Lookup Table/1, S3 Lookup Table/1, S2 Lookup Table/1, S1 Lookup Table/1
  Switch/1 -> Add/1
  Switch1/1 -> Add/2
  Switch2/1 -> Add/3
  Add/1 -> Scope/1, [Cycle]
  Constant4/1 -> Switch/3, Switch1/3, Switch2/3
  Cast To Boolean/1 -> Out1/1
  Cast To Boolean1/1 -> Out2/1
  Cast To Boolean2/1 -> Out3/1
  Cast To Boolean3/1 -> Out4/1

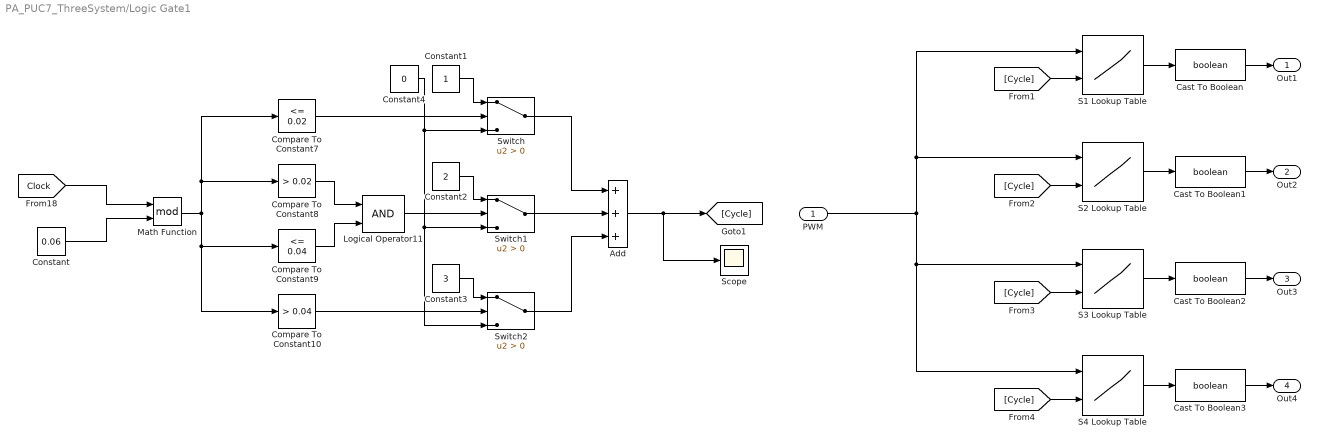
== system PA_PUC7_ThreeSystem/Logic Gate1 ==
  PWM : Inport
  Add : Sum  Inputs=+++
  Cast To Boolean{,1..3} (4 alike) : DataTypeConversion  OutDataTypeStr=boolean  SaturateOnIntegerOverflow=off  RndMeth=Floor
  Compare To Constant10 : simulink/Logic and Bit Operations/Compare To Constant  relop=>  const=0.04  OutDataTypeStr=boolean
  Compare To Constant7 : simulink/Logic and Bit Operations/Compare To Constant  relop=<=  const=0.02  OutDataTypeStr=boolean
  Compare To Constant8 : simulink/Logic and Bit Operations/Compare To Constant  relop=>  const=0.02  OutDataTypeStr=boolean
  Compare To Constant9 : simulink/Logic and Bit Operations/Compare To Constant  relop=<=  const=0.04  OutDataTypeStr=boolean
  Constant : Constant  Value=0.06
  Constant1 : Constant
  Constant2 : Constant  Value=2
  Constant3 : Constant  Value=3
  Constant4 : Constant  Value=0
  Logical Operator11 : Logic  AllPortsSameDT=off  OutDataTypeStr=boolean
  Math Function : Math  Operator=mod
  S1 Lookup Table : Lookup_n-D  BreakpointsForDimension1=[-3:3]  BreakpointsForDimension2=[1:3]  Table=[0 0 0;0 0 0;0 0 0;1 0 1;1 1 1;1 1 1;1 1 1]  InternalRulePriority=Speed  RndMeth=Simplest
      settings: InputPortMap=u0,u1
  S2 Lookup Table : Lookup_n-D  BreakpointsForDimension1=[-3:3]  BreakpointsForDimension2=[1:3]  Table=[1 1 1;1 0 1;1 0 0;1 0 1;0 1 1;0 1 0;0 0 0]  InternalRulePriority=Speed  RndMeth=Simplest
      settings: InputPortMap=u0,u1
  S3 Lookup Table : Lookup_n-D  BreakpointsForDimension1=[-3:3]  BreakpointsForDimension2=[1:3]  Table=[1 1 1;0 1 1;0 1 0;1 0 1;1 0 1;1 0 0;0 0 0]  InternalRulePriority=Speed  RndMeth=Simplest
      settings: InputPortMap=u0,u1
  S4 Lookup Table : Lookup_n-D  BreakpointsForDimension1=[-3:3]  BreakpointsForDimension2=[1:3]  Table=[1 1 1;1 1 0;0 0 1;1 0 1;1 1 0;0 0 1;0 0 0]  InternalRulePriority=Speed  RndMeth=Simplest
      settings: InputPortMap=u0,u1
  Scope : Scope
  Switch : Switch  Criteria=u2 > Threshold  SaturateOnIntegerOverflow=off  InputSameDT=off
  Switch1 : Switch  Criteria=u2 > Threshold  SaturateOnIntegerOverflow=off  InputSameDT=off
  Switch2 : Switch  Criteria=u2 > Threshold  SaturateOnIntegerOverflow=off  InputSameDT=off
  Out1 : Outport
  Out2 : Outport  Port=2
  Out3 : Outport  Port=3
  Out4 : Outport  Port=4
  wires:
  [Clock] -> Math Function/1
  Constant/1 -> Math Function/2
  Math Function/1 -> Compare To Constant7/1, Compare To Constant8/1, Compare To Constant9/1, Compare To Constant10/1
  Compare To Constant8/1 -> Logical Operator11/1
  Compare To Constant9/1 -> Logical Operator11/2
  S1 Lookup Table/1 -> Cast To Boolean/1
  S2 Lookup Table/1 -> Cast To Boolean1/1
  S3 Lookup Table/1 -> Cast To Boolean2/1
  S4 Lookup Table/1 -> Cast To Boolean3/1
  Compare To Constant7/1 -> Switch/2
  Logical Operator11/1 -> Switch1/2
  Constant1/1 -> Switch/1
  Constant2/1 -> Switch1/1
  Constant3/1 -> Switch2/1
  Compare To Constant10/1 -> Switch2/2
  [Cycle] -> S1 Lookup Table/2
  [Cycle] -> S2 Lookup Table/2
  [Cycle] -> S3 Lookup Table/2
  [Cycle] -> S4 Lookup Table/2
  PWM/1 -> S4 Lookup Table/1, S3 Lookup Table/1, S2 Lookup Table/1, S1 Lookup Table/1
  Switch/1 -> Add/1
  Switch1/1 -> Add/2
  Switch2/1 -> Add/3
  Add/1 -> Scope/1, [Cycle]
  Constant4/1 -> Switch/3, Switch1/3, Switch2/3
  Cast To Boolean/1 -> Out1/1
  Cast To Boolean1/1 -> Out2/1
  Cast To Boolean2/1 -> Out3/1
  Cast To Boolean3/1 -> Out4/1

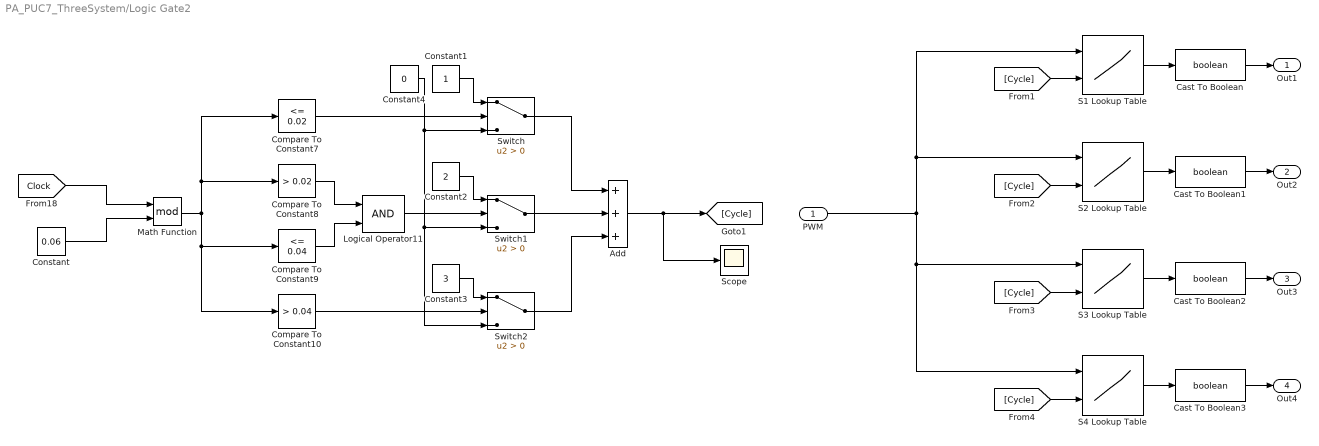
== system PA_PUC7_ThreeSystem/Logic Gate2 ==
  PWM : Inport
  Add : Sum  Inputs=+++
  Cast To Boolean{,1..3} (4 alike) : DataTypeConversion  OutDataTypeStr=boolean  SaturateOnIntegerOverflow=off  RndMeth=Floor
  Compare To Constant10 : simulink/Logic and Bit Operations/Compare To Constant  relop=>  const=0.04  OutDataTypeStr=boolean
  Compare To Constant7 : simulink/Logic and Bit Operations/Compare To Constant  relop=<=  const=0.02  OutDataTypeStr=boolean
  Compare To Constant8 : simulink/Logic and Bit Operations/Compare To Constant  relop=>  const=0.02  OutDataTypeStr=boolean
  Compare To Constant9 : simulink/Logic and Bit Operations/Compare To Constant  relop=<=  const=0.04  OutDataTypeStr=boolean
  Constant : Constant  Value=0.06
  Constant1 : Constant
  Constant2 : Constant  Value=2
  Constant3 : Constant  Value=3
  Constant4 : Constant  Value=0
  Logical Operator11 : Logic  AllPortsSameDT=off  OutDataTypeStr=boolean
  Math Function : Math  Operator=mod
  S1 Lookup Table : Lookup_n-D  BreakpointsForDimension1=[-3:3]  BreakpointsForDimension2=[1:3]  Table=[0 0 0;0 0 0;0 0 0;1 0 1;1 1 1;1 1 1;1 1 1]  InternalRulePriority=Speed  RndMeth=Simplest
      settings: InputPortMap=u0,u1
  S2 Lookup Table : Lookup_n-D  BreakpointsForDimension1=[-3:3]  BreakpointsForDimension2=[1:3]  Table=[1 1 1;1 0 1;1 0 0;1 0 1;0 1 1;0 1 0;0 0 0]  InternalRulePriority=Speed  RndMeth=Simplest
      settings: InputPortMap=u0,u1
  S3 Lookup Table : Lookup_n-D  BreakpointsForDimension1=[-3:3]  BreakpointsForDimension2=[1:3]  Table=[1 1 1;0 1 1;0 1 0;1 0 1;1 0 1;1 0 0;0 0 0]  InternalRulePriority=Speed  RndMeth=Simplest
      settings: InputPortMap=u0,u1
  S4 Lookup Table : Lookup_n-D  BreakpointsForDimension1=[-3:3]  BreakpointsForDimension2=[1:3]  Table=[1 1 1;1 1 0;0 0 1;1 0 1;1 1 0;0 0 1;0 0 0]  InternalRulePriority=Speed  RndMeth=Simplest
      settings: InputPortMap=u0,u1
  Scope : Scope
  Switch : Switch  Criteria=u2 > Threshold  SaturateOnIntegerOverflow=off  InputSameDT=off
  Switch1 : Switch  Criteria=u2 > Threshold  SaturateOnIntegerOverflow=off  InputSameDT=off
  Switch2 : Switch  Criteria=u2 > Threshold  SaturateOnIntegerOverflow=off  InputSameDT=off
  Out1 : Outport
  Out2 : Outport  Port=2
  Out3 : Outport  Port=3
  Out4 : Outport  Port=4
  wires:
  [Clock] -> Math Function/1
  Constant/1 -> Math Function/2
  Math Function/1 -> Compare To Constant7/1, Compare To Constant8/1, Compare To Constant9/1, Compare To Constant10/1
  Compare To Constant8/1 -> Logical Operator11/1
  Compare To Constant9/1 -> Logical Operator11/2
  S1 Lookup Table/1 -> Cast To Boolean/1
  S2 Lookup Table/1 -> Cast To Boolean1/1
  S3 Lookup Table/1 -> Cast To Boolean2/1
  S4 Lookup Table/1 -> Cast To Boolean3/1
  Compare To Constant7/1 -> Switch/2
  Logical Operator11/1 -> Switch1/2
  Constant1/1 -> Switch/1
  Constant2/1 -> Switch1/1
  Constant3/1 -> Switch2/1
  Compare To Constant10/1 -> Switch2/2
  [Cycle] -> S1 Lookup Table/2
  [Cycle] -> S2 Lookup Table/2
  [Cycle] -> S3 Lookup Table/2
  [Cycle] -> S4 Lookup Table/2
  PWM/1 -> S4 Lookup Table/1, S3 Lookup Table/1, S2 Lookup Table/1, S1 Lookup Table/1
  Switch/1 -> Add/1
  Switch1/1 -> Add/2
  Switch2/1 -> Add/3
  Add/1 -> Scope/1, [Cycle]
  Constant4/1 -> Switch/3, Switch1/3, Switch2/3
  Cast To Boolean/1 -> Out1/1
  Cast To Boolean1/1 -> Out2/1
  Cast To Boolean2/1 -> Out3/1
  Cast To Boolean3/1 -> Out4/1

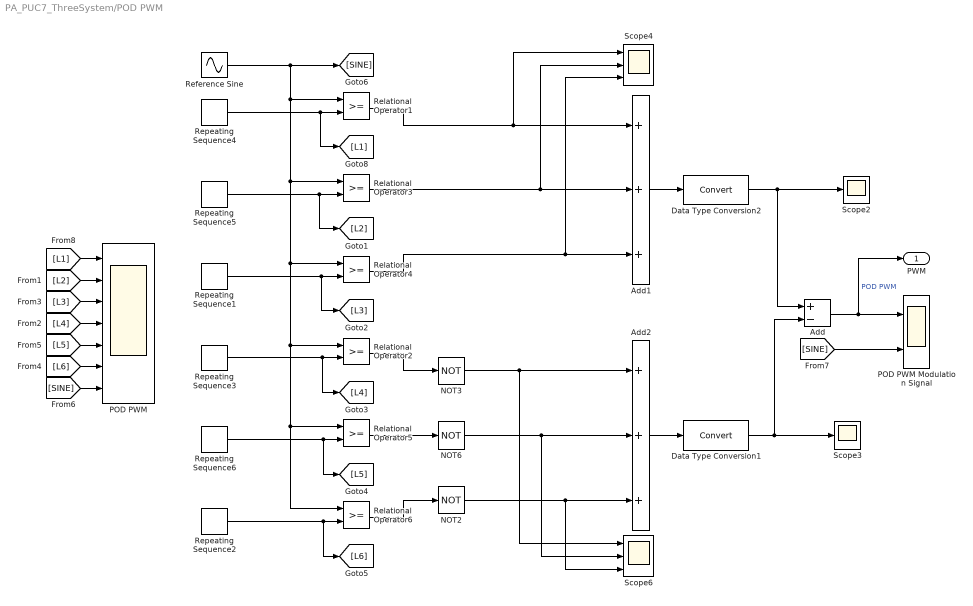
== system PA_PUC7_ThreeSystem/POD PWM ==
  Add : Sum  Inputs=+-
  Add1 : Sum  Inputs=+++
  Add2 : Sum  Inputs=+++
  Data Type Conversion1 : DataTypeConversion  SaturateOnIntegerOverflow=off  RndMeth=Floor
  Data Type Conversion2 : DataTypeConversion  SaturateOnIntegerOverflow=off  RndMeth=Floor
  NOT2 : Logic  Operator=NOT  AllPortsSameDT=off  OutDataTypeStr=boolean
  NOT3 : Logic  Operator=NOT  AllPortsSameDT=off  OutDataTypeStr=boolean
  NOT6 : Logic  Operator=NOT  AllPortsSameDT=off  OutDataTypeStr=boolean
  POD PWM : Scope  NumInputPorts=7
  POD PWM Modulation Signal : Scope  NumInputPorts=2
  Reference Sine : Sin  Amplitude=3  Frequency=2*pi*50  Phase=2*pi*(3/4)  SampleTime=0
  Relational Operator{1..6} (6 alike) : RelationalOperator  OutDataTypeStr=boolean  InputSameDT=off
  Repeating Sequence1 : simulink/Sources/Repeating Sequence  rep_seq_t=[0 0.5 1]/2500  rep_seq_y="[1  0  1]"
  Repeating Sequence2 : simulink/Sources/Repeating Sequence  rep_seq_t=[0 0.5 1]/2500  rep_seq_y="[-3  -2  -3]"
  Repeating Sequence3 : simulink/Sources/Repeating Sequence  rep_seq_t=[0 0.5 1]/2500  rep_seq_y=[-1 0 -1]
  Repeating Sequence4 : simulink/Sources/Repeating Sequence  rep_seq_t=[0 0.5 1]/2500  rep_seq_y=[3 2 3]
  Repeating Sequence5 : simulink/Sources/Repeating Sequence  rep_seq_t=[0 0.5 1]/2500  rep_seq_y="[2  1  2]"
  Repeating Sequence6 : simulink/Sources/Repeating Sequence  rep_seq_t=[0 0.5 1]/2500  rep_seq_y="[-2  -1  -2]"
  Scope2 : Scope
  Scope3 : Scope
  Scope4 : Scope  NumInputPorts=3
  Scope6 : Scope  NumInputPorts=3
  PWM : Outport
  wires:
  Repeating Sequence5/1 -> [L2], Relational Operator3/2
  Reference Sine/1 -> [SINE], Relational Operator2/1, Relational Operator6/1, Relational Operator5/1, Relational Operator4/1, Relational Operator3/1, Relational Operator1/1
  Repeating Sequence4/1 -> [L1], Relational Operator1/2
  Relational Operator1/1 -> Scope4/1, Add1/1
  Relational Operator3/1 -> Scope4/2, Add1/2
  Repeating Sequence1/1 -> [L3], Relational Operator4/2
  Relational Operator4/1 -> Scope4/3, Add1/3
  Repeating Sequence3/1 -> [L4], Relational Operator2/2
  Relational Operator6/1 -> NOT2/1
  Repeating Sequence6/1 -> [L5], Relational Operator5/2
  Repeating Sequence2/1 -> [L6], Relational Operator6/2
  Relational Operator2/1 -> NOT3/1
  Relational Operator5/1 -> NOT6/1
  [L1] -> POD PWM/1
  [L2] -> POD PWM/2
  [L5] -> POD PWM/5
  [L3] -> POD PWM/3
  [L4] -> POD PWM/4
  [L6] -> POD PWM/6
  [SINE] -> POD PWM/7
  Add/1 -> PWM/1, POD PWM Modulation Signal/1  "POD PWM"
  [SINE] -> POD PWM Modulation Signal/2
  NOT2/1 -> Scope6/3, Add2/3
  Add2/1 -> Data Type Conversion1/1
  Add1/1 -> Data Type Conversion2/1
  Data Type Conversion2/1 -> Scope2/1, Add/1
  Data Type Conversion1/1 -> Scope3/1, Add/2
  NOT6/1 -> Add2/2, Scope6/2
  NOT3/1 -> Scope6/1, Add2/1

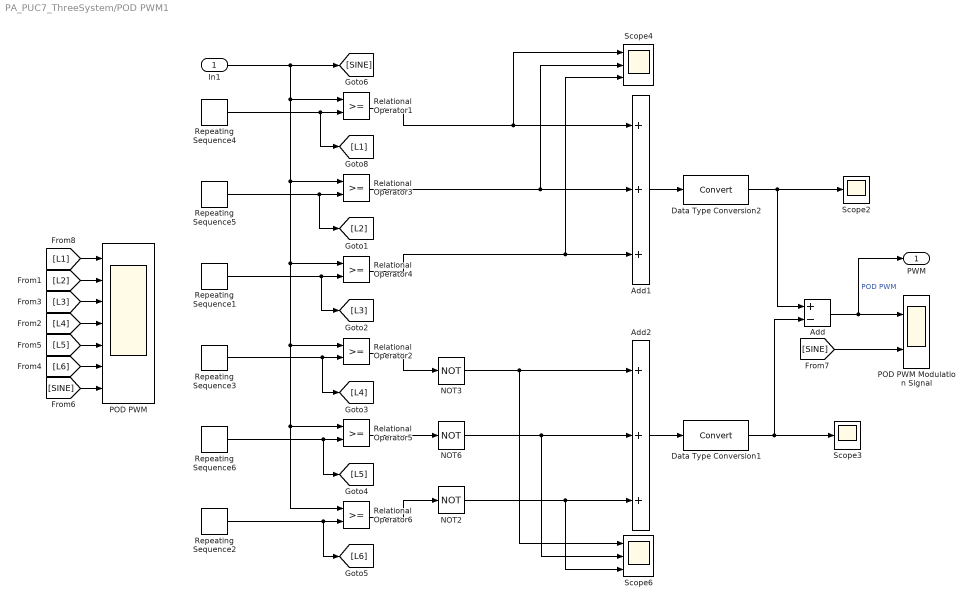
== system PA_PUC7_ThreeSystem/POD PWM1 ==
  In1 : Inport
  Add : Sum  Inputs=+-
  Add1 : Sum  Inputs=+++
  Add2 : Sum  Inputs=+++
  Data Type Conversion1 : DataTypeConversion  SaturateOnIntegerOverflow=off  RndMeth=Floor
  Data Type Conversion2 : DataTypeConversion  SaturateOnIntegerOverflow=off  RndMeth=Floor
  NOT2 : Logic  Operator=NOT  AllPortsSameDT=off  OutDataTypeStr=boolean
  NOT3 : Logic  Operator=NOT  AllPortsSameDT=off  OutDataTypeStr=boolean
  NOT6 : Logic  Operator=NOT  AllPortsSameDT=off  OutDataTypeStr=boolean
  POD PWM : Scope  NumInputPorts=7
  POD PWM Modulation Signal : Scope  NumInputPorts=2
  Relational Operator{1..6} (6 alike) : RelationalOperator  OutDataTypeStr=boolean  InputSameDT=off
  Repeating Sequence1 : simulink/Sources/Repeating Sequence  rep_seq_t=[0 0.5 1]/2500  rep_seq_y="[1  0  1]"
  Repeating Sequence2 : simulink/Sources/Repeating Sequence  rep_seq_t=[0 0.5 1]/2500  rep_seq_y="[-3  -2  -3]"
  Repeating Sequence3 : simulink/Sources/Repeating Sequence  rep_seq_t=[0 0.5 1]/2500  rep_seq_y=[-1 0 -1]
  Repeating Sequence4 : simulink/Sources/Repeating Sequence  rep_seq_t=[0 0.5 1]/2500  rep_seq_y=[3 2 3]
  Repeating Sequence5 : simulink/Sources/Repeating Sequence  rep_seq_t=[0 0.5 1]/2500  rep_seq_y="[2  1  2]"
  Repeating Sequence6 : simulink/Sources/Repeating Sequence  rep_seq_t=[0 0.5 1]/2500  rep_seq_y="[-2  -1  -2]"
  Scope2 : Scope
  Scope3 : Scope
  Scope4 : Scope  NumInputPorts=3
  Scope6 : Scope  NumInputPorts=3
  PWM : Outport
  wires:
  Repeating Sequence5/1 -> [L2], Relational Operator3/2
  In1/1 -> [SINE], Relational Operator2/1, Relational Operator6/1, Relational Operator5/1, Relational Operator4/1, Relational Operator3/1, Relational Operator1/1
  Repeating Sequence4/1 -> [L1], Relational Operator1/2
  Relational Operator1/1 -> Scope4/1, Add1/1
  Relational Operator3/1 -> Scope4/2, Add1/2
  Repeating Sequence1/1 -> [L3], Relational Operator4/2
  Relational Operator4/1 -> Scope4/3, Add1/3
  Repeating Sequence3/1 -> [L4], Relational Operator2/2
  Relational Operator6/1 -> NOT2/1
  Repeating Sequence6/1 -> [L5], Relational Operator5/2
  Repeating Sequence2/1 -> [L6], Relational Operator6/2
  Relational Operator2/1 -> NOT3/1
  Relational Operator5/1 -> NOT6/1
  [L1] -> POD PWM/1
  [L2] -> POD PWM/2
  [L5] -> POD PWM/5
  [L3] -> POD PWM/3
  [L4] -> POD PWM/4
  [L6] -> POD PWM/6
  [SINE] -> POD PWM/7
  Add/1 -> PWM/1, POD PWM Modulation Signal/1  "POD PWM"
  [SINE] -> POD PWM Modulation Signal/2
  NOT2/1 -> Scope6/3, Add2/3
  Add2/1 -> Data Type Conversion1/1
  Add1/1 -> Data Type Conversion2/1
  Data Type Conversion2/1 -> Scope2/1, Add/1
  Data Type Conversion1/1 -> Scope3/1, Add/2
  NOT6/1 -> Add2/2, Scope6/2
  NOT3/1 -> Scope6/1, Add2/1

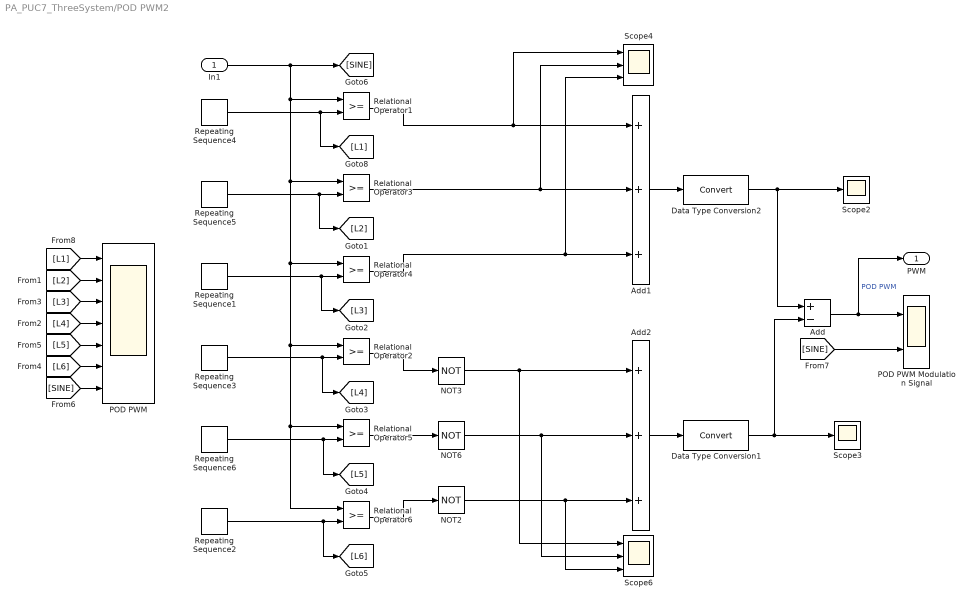
== system PA_PUC7_ThreeSystem/POD PWM2 ==
  In1 : Inport
  Add : Sum  Inputs=+-
  Add1 : Sum  Inputs=+++
  Add2 : Sum  Inputs=+++
  Data Type Conversion1 : DataTypeConversion  SaturateOnIntegerOverflow=off  RndMeth=Floor
  Data Type Conversion2 : DataTypeConversion  SaturateOnIntegerOverflow=off  RndMeth=Floor
  NOT2 : Logic  Operator=NOT  AllPortsSameDT=off  OutDataTypeStr=boolean
  NOT3 : Logic  Operator=NOT  AllPortsSameDT=off  OutDataTypeStr=boolean
  NOT6 : Logic  Operator=NOT  AllPortsSameDT=off  OutDataTypeStr=boolean
  POD PWM : Scope  NumInputPorts=7
  POD PWM Modulation Signal : Scope  NumInputPorts=2
  Relational Operator{1..6} (6 alike) : RelationalOperator  OutDataTypeStr=boolean  InputSameDT=off
  Repeating Sequence1 : simulink/Sources/Repeating Sequence  rep_seq_t=[0 0.5 1]/2500  rep_seq_y="[1  0  1]"
  Repeating Sequence2 : simulink/Sources/Repeating Sequence  rep_seq_t=[0 0.5 1]/2500  rep_seq_y="[-3  -2  -3]"
  Repeating Sequence3 : simulink/Sources/Repeating Sequence  rep_seq_t=[0 0.5 1]/2500  rep_seq_y=[-1 0 -1]
  Repeating Sequence4 : simulink/Sources/Repeating Sequence  rep_seq_t=[0 0.5 1]/2500  rep_seq_y=[3 2 3]
  Repeating Sequence5 : simulink/Sources/Repeating Sequence  rep_seq_t=[0 0.5 1]/2500  rep_seq_y="[2  1  2]"
  Repeating Sequence6 : simulink/Sources/Repeating Sequence  rep_seq_t=[0 0.5 1]/2500  rep_seq_y="[-2  -1  -2]"
  Scope2 : Scope
  Scope3 : Scope
  Scope4 : Scope  NumInputPorts=3
  Scope6 : Scope  NumInputPorts=3
  PWM : Outport
  wires:
  Repeating Sequence5/1 -> [L2], Relational Operator3/2
  In1/1 -> [SINE], Relational Operator2/1, Relational Operator6/1, Relational Operator5/1, Relational Operator4/1, Relational Operator3/1, Relational Operator1/1
  Repeating Sequence4/1 -> [L1], Relational Operator1/2
  Relational Operator1/1 -> Scope4/1, Add1/1
  Relational Operator3/1 -> Scope4/2, Add1/2
  Repeating Sequence1/1 -> [L3], Relational Operator4/2
  Relational Operator4/1 -> Scope4/3, Add1/3
  Repeating Sequence3/1 -> [L4], Relational Operator2/2
  Relational Operator6/1 -> NOT2/1
  Repeating Sequence6/1 -> [L5], Relational Operator5/2
  Repeating Sequence2/1 -> [L6], Relational Operator6/2
  Relational Operator2/1 -> NOT3/1
  Relational Operator5/1 -> NOT6/1
  [L1] -> POD PWM/1
  [L2] -> POD PWM/2
  [L5] -> POD PWM/5
  [L3] -> POD PWM/3
  [L4] -> POD PWM/4
  [L6] -> POD PWM/6
  [SINE] -> POD PWM/7
  Add/1 -> PWM/1, POD PWM Modulation Signal/1  "POD PWM"
  [SINE] -> POD PWM Modulation Signal/2
  NOT2/1 -> Scope6/3, Add2/3
  Add2/1 -> Data Type Conversion1/1
  Add1/1 -> Data Type Conversion2/1
  Data Type Conversion2/1 -> Scope2/1, Add/1
  Data Type Conversion1/1 -> Scope3/1, Add/2
  NOT6/1 -> Add2/2, Scope6/2
  NOT3/1 -> Scope6/1, Add2/1

== matlab function PA_PUC7_ThreeSystem/MATLAB Function ==
  data: t input; R output
function R = time_dependent_R(t)
    if t < 4
        R = 100;
    elseif t < 5.5
        R = 500;
    else
        R = 100;
    end
end
